simulink model "mehmet"  (R2017b)
settings: Solver=VariableStepAuto  StartTime=0.0  StopTime=5  MaxStep=0.001  RelTol=1e-3
settings Model: Creator=user  LastModifiedBy=user

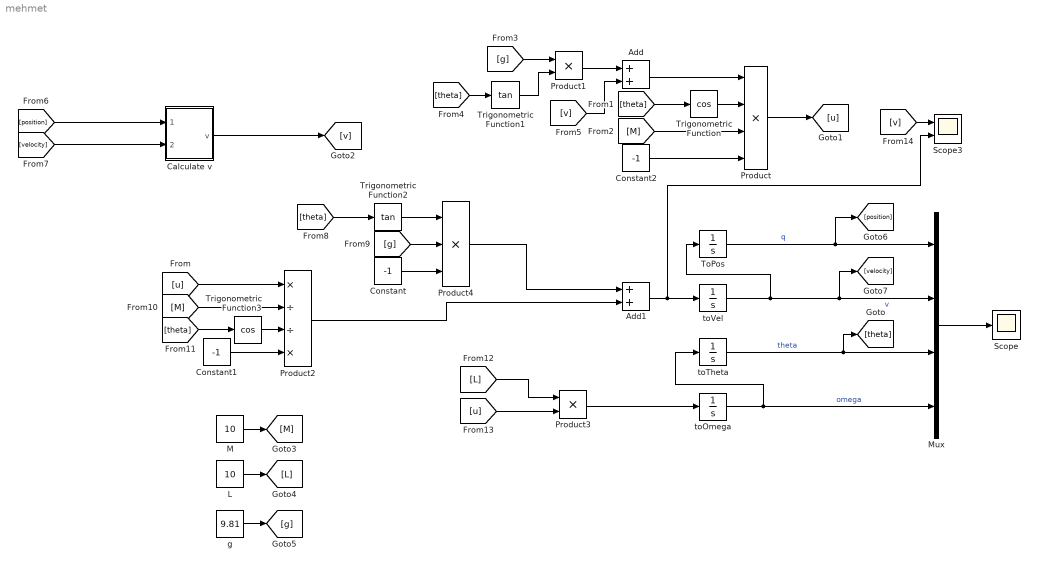
== system mehmet ==
  Add : Sum
  Add1 : Sum
  Calculate v : Subsystem
  Constant : Constant  Value=-1
  Constant1 : Constant  Value=-1
  Constant2 : Constant  Value=-1
  L : Constant  Value=10
  M : Constant  Value=10
  Mux : Mux
  Product : Product  Inputs=4
  Product1 : Product
  Product2 : Product  Inputs=*//*
  Product3 : Product
  Product4 : Product  Inputs=3
  Scope : Scope
  Scope3 : Scope  NumInputPorts=2
  ToPos : Integrator  InitialCondition=1
  Trigonometric Function : Trigonometry  Operator=cos
  Trigonometric Function1 : Trigonometry  Operator=tan
  Trigonometric Function2 : Trigonometry  Operator=tan
  Trigonometric Function3 : Trigonometry  Operator=cos
  g : Constant  Value=9.81
  toOmega : Integrator
  toTheta : Integrator
  toVel : Integrator
  wires:
  toVel/1 -> ToPos/1, [velocity], Mux/2  "v"
  ToPos/1 -> [position], Mux/1  "q"
  toOmega/1 -> Mux/4, toTheta/1  "omega"
  toTheta/1 -> Mux/3, [theta]  "theta"
  Trigonometric Function/1 -> Product/2
  [theta] -> Trigonometric Function/1
  M/1 -> [M]
  [M] -> Product/3
  L/1 -> [L]
  g/1 -> [g]
  [theta] -> Trigonometric Function1/1
  [g] -> Product1/1
  Trigonometric Function1/1 -> Product1/2
  Product1/1 -> Add/1
  [v] -> Add/2
  Add/1 -> Product/1
  Product/1 -> [u]
  [theta] -> Trigonometric Function2/1
  Trigonometric Function2/1 -> Product4/1
  Constant/1 -> Product4/3
  [g] -> Product4/2
  [position] -> Calculate v/1(position)
  [velocity] -> Calculate v/2("velocity ")
  Calculate v/1(v) -> [v]
  [u] -> Product2/1
  [M] -> Product2/2
  [theta] -> Trigonometric Function3/1
  Trigonometric Function3/1 -> Product2/3
  Constant1/1 -> Product2/4
  Product4/1 -> Add1/1
  Product2/1 -> Add1/2
  Add1/1 -> Scope3/2, toVel/1
  [u] -> Product3/2
  [L] -> Product3/1
  Product3/1 -> toOmega/1
  Mux/1 -> Scope/1
  [v] -> Scope3/1
  Constant2/1 -> Product/4

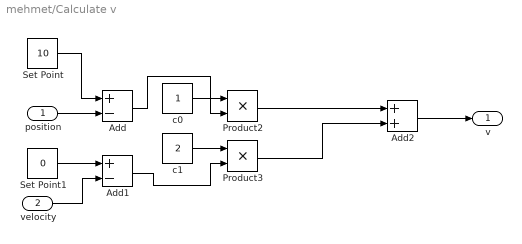
== system mehmet/Calculate v ==
  position : Inport
  "velocity " : Inport  Port=2
  Add : Sum  Inputs=+-
  Add1 : Sum  Inputs=+-
  Add2 : Sum
  Product2 : Product
  Product3 : Product
  Set Point : Constant  Value=10
  Set Point1 : Constant  Value=0
  c0 : Constant
  c1 : Constant  Value=2
  v : Outport
  wires:
  c1/1 -> Product3/1
  c0/1 -> Product2/1
  Add2/1 -> v/1
  Product2/1 -> Add2/1
  Product3/1 -> Add2/2
  Set Point/1 -> Add/1
  position/1 -> Add/2
  Add/1 -> Product2/2
  Set Point1/1 -> Add1/1
  "velocity "/1 -> Add1/2
  Add1/1 -> Product3/2
